simulink library "INT_ACCmpr_VD"  (R2016b)
settings: Solver=VariableStepAuto  StartTime=0.0  StopTime=10.0  RelTol=1e-3
settings Model: Creator=lenovo  LastModifiedBy=lenovo

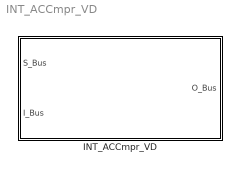
== system INT_ACCmpr_VD ==
  INT_ACCmpr_VD : Subsystem

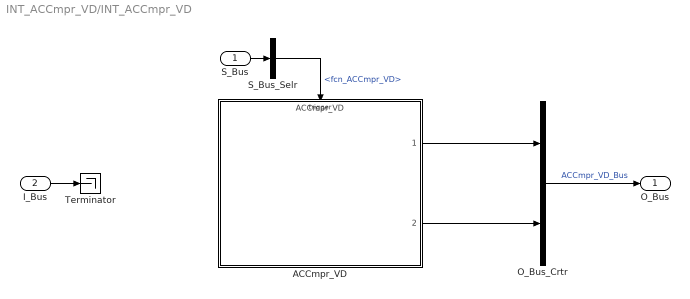
== system INT_ACCmpr_VD/INT_ACCmpr_VD ==
  S_Bus : Inport
  I_Bus : Inport  Port=2
  ACCmpr_VD : ModelReference  ModelNameDialog=ACCmpr_VD  SimulationMode=Normal  ModelReferenceVersion=1.9  TriggerPortName=function  TriggerPortTriggerType=function-call  TriggerPortStatesWhenEnabling=held
  O_Bus_Crtr : BusCreator  Inputs=2
  S_Bus_Selr : BusSelector  OutputSignals=fcn_ACCmpr_VD
  Terminator : Terminator
  O_Bus : Outport
  wires:
  S_Bus_Selr/1 -> ACCmpr_VD/Trigger  "<fcn_ACCmpr_VD>"
  S_Bus/1 -> S_Bus_Selr/1
  I_Bus/1 -> Terminator/1
  O_Bus_Crtr/1 -> O_Bus/1  "ACCmpr_VD_Bus"
  ACCmpr_VD/1 -> O_Bus_Crtr/1
  ACCmpr_VD/2 -> O_Bus_Crtr/2
